simulink model "nucleo_f446_CR12832"  (R2015a)
settings: Solver=ode45  StartTime=0.0  StopTime=10.0  RelTol=1e-3
libraries: mbed_spi_several x1
settings Model: Creator=oh  LastModifiedBy=oh

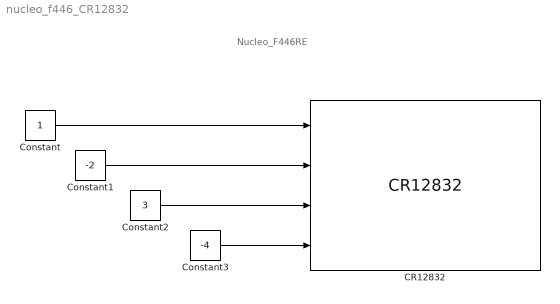
== system nucleo_f446_CR12832 ==
  note: Nucleo_F446RE
  CR12832 : mbed_spi_several/CR12832  TypeOfInputs1={'uint8' 'int8'}  NumberOfInputs1=2  Row1='row1 %hu %hd'  TypeOfInputs2={'single'}  NumberOfInputs2=1  Row2='row2 %f'  TypeOfInputs3={'int32'}  NumberOfInputs3=1  Row3='row3 %lf'  SpiPort=1  CsPort=A  CsPin=0  ResPort=A  ResPin=0  A0Port=A  A0Pin=0  SampleTime=-1
  Constant : Constant  OutDataTypeStr=Inherit: Inherit via back propagation
  Constant1 : Constant  Value=-2  OutDataTypeStr=Inherit: Inherit via back propagation
  Constant2 : Constant  Value=3  OutDataTypeStr=Inherit: Inherit via back propagation
  Constant3 : Constant  Value=-4  OutDataTypeStr=Inherit: Inherit via back propagation
  wires:
  Constant/1 -> CR12832/1
  Constant1/1 -> CR12832/2
  Constant2/1 -> CR12832/3
  Constant3/1 -> CR12832/4
